simulink model "regulator_opt"  (R2019b)
settings: Solver=VariableStepAuto  StartTime=0.0  StopTime=10  RelTol=1e-3
values from neighbouring files (symbols this model uses):
  a = param_set(5)    [eom.m]    (also in main.m = 0.005; reduced_pressure.m)
  A_o2 = param_set(1)    [eom.m]    (also in main.m = 7.85398163397e-07; reduced_pressure.m)
  beta_o2 = param_set(2)    [eom.m]    (also in main.m = 0.25; reduced_pressure.m)
  k = param_set(8)    [eom.m]    (also in main.m = 2300)
  m_s = param_set(9)    [eom.m]    (also in main.m = spool_mass(a); spool_mass.m = V_s*rho)
  P_des = 1e6    (= 1000000)    [main.m]
  P_out = param_set(3)    [eom.m]    (also in main.m = 0; reduced_pressure.m)
undefined symbols (not defined in the file or in its folder): sigbuilder_block
settings Model: Creator=Alexander  LastModifiedBy=Alexander

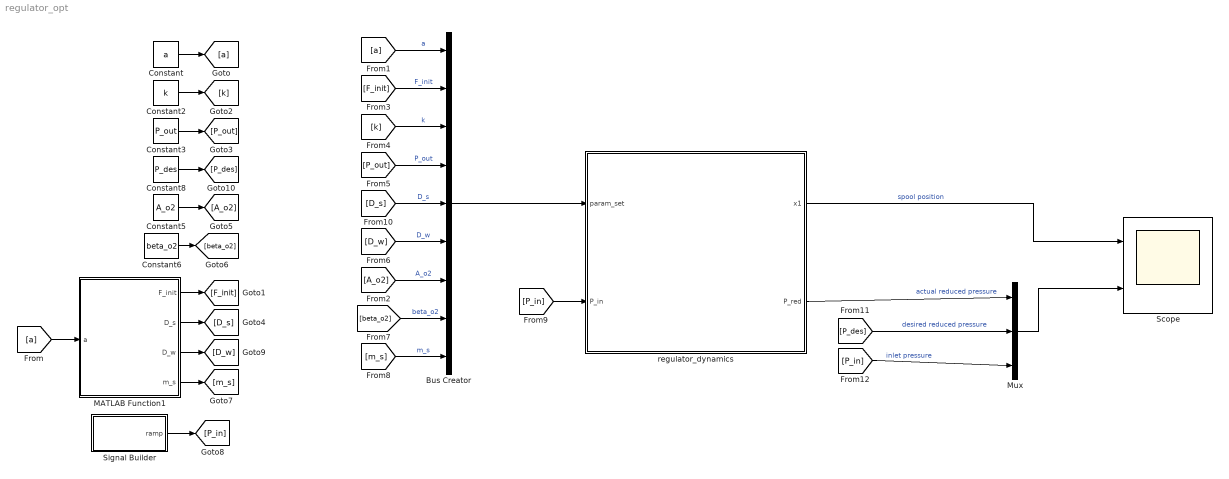
== system regulator_opt ==
  Bus Creator : BusCreator  Inputs=9
  Constant : Constant  Value=a
  Constant2 : Constant  Value=k
  Constant3 : Constant  Value=P_out
  Constant5 : Constant  Value=A_o2
  Constant6 : Constant  Value=beta_o2
  Constant8 : Constant  Value=P_des
  MATLAB Function1 : MATLAB Function  TreatAsAtomicUnit=on
  Mux : Mux  Inputs=3
  Scope : Scope  NumInputPorts=2
  Signal Builder : Subsystem  Tag=STV Subsys  LoadFcn=sigbuilder_block('load');  StartFcn=sigbuilder_block('start');  StopFcn=sigbuilder_block('stop');  ClipboardFcn=sigbuilder_block('clipboard');  mask(Sigbuilder block){tuvar=[0:10]}
      mask help: Simulink:masks:SigbuilderBlock_MD
      mask init:
      | if ~strcmp(get_param(bdroot(gcbh),'SimulationStatus'),'stopped') tuvar = sigbuilder_block('maskInit'); end
      settings: CopyFcn=sigbuilder_block('copy');  DeleteFcn=sigbuilder_block('delete');  ModelCloseFcn=sigbuilder_block('modelClose');  PreSaveFcn=sigbuilder_block('preSave');  PauseFcn=sigbuilder_block('pause');  ContinueFcn=sigbuilder_block('continue');  NameChangeFcn=sigbuilder_block('namechange');  OpenFcn=sigbuilder_block('open',[437.6 199.2 550.4 400 ]);  CloseFcn=sigbuilder_block('close');
      mask Display: plot(0, 0, 100, 100,[2, 2, 32, 32, 2], [68, 8, 8, 68, 68],[32, 2], [38, 38], [32, 19, 2],[53, 60, 44], [32, 17, 17, 2],[16, 16, 31, 31]);txt = getActiveGroup(gcbh);text(2, 100, txt,'verticalAlignment', 'top');
  regulator_dynamics : Subsystem
  wires:
  Constant/1 -> [a]
  Constant2/1 -> [k]
  Constant3/1 -> [P_out]
  Constant5/1 -> [A_o2]
  Constant6/1 -> [beta_o2]
  [a] -> MATLAB Function1/1(a)
  MATLAB Function1/4(m_s) -> [m_s]
  [a] -> Bus Creator/1  "a"
  [m_s] -> Bus Creator/9  "m_s"
  [F_init] -> Bus Creator/2  "F_init"
  [k] -> Bus Creator/3  "k"
  [D_w] -> Bus Creator/6  "D_w"
  [A_o2] -> Bus Creator/7  "A_o2"
  [beta_o2] -> Bus Creator/8  "beta_o2"
  Bus Creator/1 -> regulator_dynamics/1(param_set)
  regulator_dynamics/2(P_red) -> Mux/1  "actual reduced pressure"
  Signal Builder/1(ramp) -> [P_in]
  [P_in] -> regulator_dynamics/2(P_in)
  [P_out] -> Bus Creator/4  "P_out"
  [D_s] -> Bus Creator/5  "D_s"
  Constant8/1 -> [P_des]
  [P_des] -> Mux/2  "desired reduced pressure"
  [P_in] -> Mux/3  "inlet pressure"
  regulator_dynamics/1(x1) -> Scope/1  "spool position"
  Mux/1 -> Scope/2
  MATLAB Function1/1(F_init) -> [F_init]
  MATLAB Function1/2(D_s) -> [D_s]
  MATLAB Function1/3(D_w) -> [D_w]

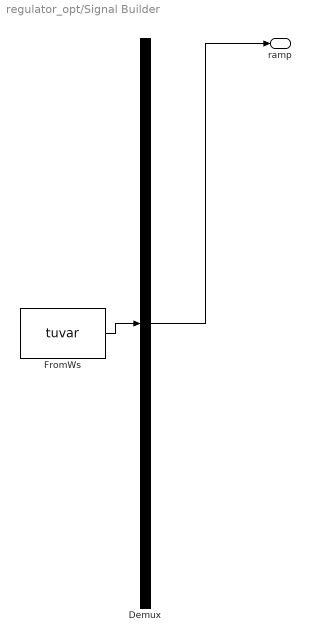
== system regulator_opt/Signal Builder ==
  Demux : Demux  Tag=STV Demux  Outputs=1
  FromWs : FromWorkspace  Tag=STV FromWs  VariableName=tuvar  SampleTime=0
      SigBuilderData=|
      | common.afterFinalStr = 'Extrapolate'
      | common.sampleTime = 0
      | dataSet.timeRange = [0 10]
      | dataSet.name = 'inlet_pressure'
      | sbobj.Groups.Name = 'inlet_pressure'
      | sbobj.Groups.Signals.Name = 'ramp'
      | sbobj.Groups.Signals.XData = [0 10]
      | sbobj.Groups.Signals.YData = [100000 2000000]
  ramp : Outport  Tag=STV Outport
  wires:
  Demux/1 -> ramp/1
  FromWs/1 -> Demux/1

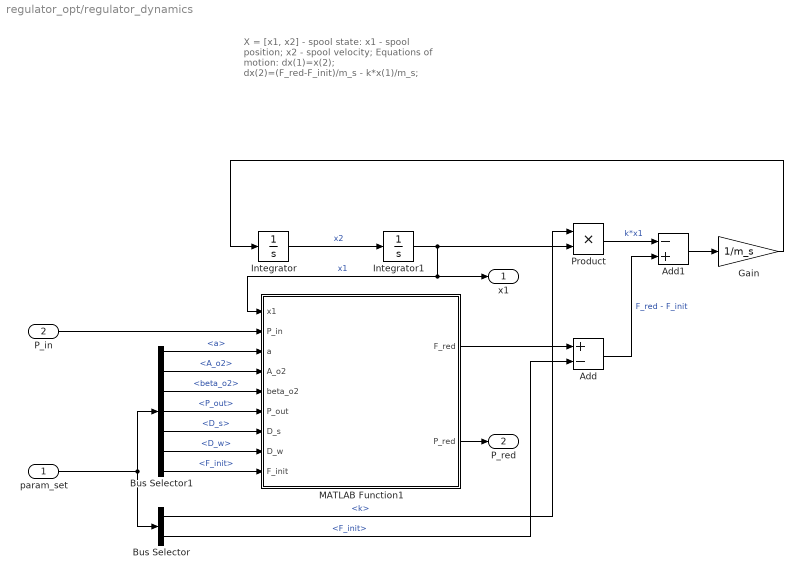
== system regulator_opt/regulator_dynamics ==
  note: X = [x1, x2] - spool state:
      | 	x1 - spool position;
      | 	x2 - spool velocity;
      |
      | Equations of motion:
      | dx(1)=x(2);
      | dx(2)=(F_red-F_init)/m_s - k*x(1)/m_s;
  param_set : Inport
  P_in : Inport  Port=2
  Add : Sum  Inputs=+-
  Add1 : Sum  Inputs=-+
  Bus Selector : BusSelector  OutputSignals=k,F_init
  Bus Selector1 : BusSelector  OutputSignals=a,A_o2,beta_o2,P_out,D_s,D_w,F_init
  Gain : Gain  Gain=1/m_s
  Integrator : Integrator
  Integrator1 : Integrator
  MATLAB Function1 : MATLAB Function  TreatAsAtomicUnit=on
  Product : Product
  x1 : Outport
  P_red : Outport  Port=2
  wires:
  MATLAB Function1/2(P_red) -> P_red/1
  P_in/1 -> MATLAB Function1/2(P_in)
  Add/1 -> Add1/2  "F_red - F_init"
  MATLAB Function1/1(F_red) -> Add/1
  Integrator/1 -> Integrator1/1  "x2"
  Product/1 -> Add1/1  "k*x1"
  Gain/1 -> Integrator/1
  Add1/1 -> Gain/1
  param_set/1 -> Bus Selector/1, Bus Selector1/1
  Bus Selector/1 -> Product/1  "<k>"
  Bus Selector/2 -> Add/2  "<F_init>"
  Integrator1/1 -> Product/2, MATLAB Function1/1(x1), x1/1  "x1"
  Bus Selector1/7 -> MATLAB Function1/9(F_init)  "<F_init>"
  Bus Selector1/6 -> MATLAB Function1/8(D_w)  "<D_w>"
  Bus Selector1/5 -> MATLAB Function1/7(D_s)  "<D_s>"
  Bus Selector1/4 -> MATLAB Function1/6(P_out)  "<P_out>"
  Bus Selector1/3 -> MATLAB Function1/5(beta_o2)  "<beta_o2>"
  Bus Selector1/2 -> MATLAB Function1/4(A_o2)  "<A_o2>"
  Bus Selector1/1 -> MATLAB Function1/3(a)  "<a>"

== matlab function regulator_opt/regulator_dynamics/MATLAB Function1 ==
  data: x1 input; F_red output; P_in input; a input; A_o2 input; P_red output; beta_o2 input; P_out input; D_s input; D_w input; F_init input
function [F_red, P_red]  = reduced_pressure_force(x1, P_in, a, ...
                            A_o2, beta_o2, P_out, D_s, D_w, F_init)
% current reduced pressure force calculation
%%
% calculate reduced pressure
A_o1 = a*(a-x1);                    % current area of the valve

if A_o1<0, A_o1 = 0;
end                                 % valve closes if x(1)>a, so A_o1 is non-negative

beta_o1 = sqrt(4*A_o1/pi)/D_w;      % current area of the valve/pipe

gamma_1 = A_o1*(1-beta_o2^4);
gamma_2 = A_o2*(1-beta_o1^4);
% calculate current reduced pressure
P_red = (gamma_1*P_in + gamma_2*P_out)/(gamma_1 + gamma_2);
% and reduced pressure force on the spool, assuming it acts on the whole
% surface, i.e. shoulder area is neglected (unlike the shoulder force)
% only gauge pressure generates force, hence the P_red-Pout term

F_red = (P_red-P_out)*(pi*D_s^2)/4;

if F_red<F_init
    F_red = F_init;
end
end

== matlab function regulator_opt/MATLAB Function1 ==
  data: F_init output; a input; D_s output; D_w output; m_s output
function [F_init, D_s, D_w, m_s] = param_init(a)
% function initializes all parameters that depend on the variable
% parameters of the window size 'a' 
%%
D_s = 3*a;                              % spool diameter
F_init = 1e6*(pi*D_s^2)/4;              % initial force on the spool
D_w = sqrt(4*a^2/pi);                   % equivalent diameter of the window

% calculate spool volume
V_s = 2*a*(pi*(3*a)^2)/4 + a*(pi*(1.5*a)^2)/4;

% calculate spool mass
rho = 7.8e3;
m_s = V_s*rho;
